simulink model "ecg_simulation"  (R2024b)
settings: Solver=VariableStepAuto  StartTime=0.0  StopTime=10.0  RelTol=1e-3
libraries: simulink x1

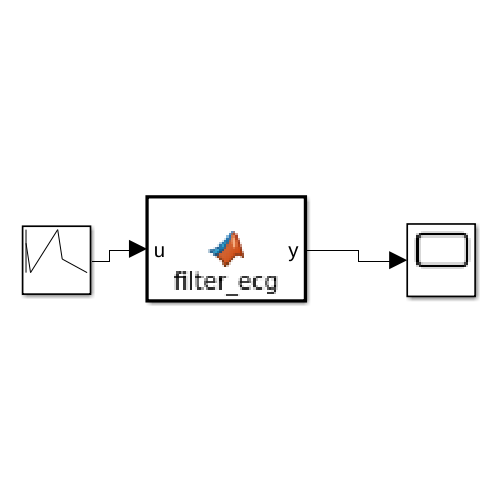
[thumbnail: Simulink's stored preview of the top-level diagram]
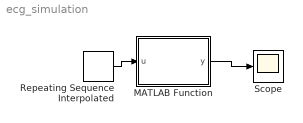
== system ecg_simulation ==
  MATLAB Function : MATLAB Function  TreatAsAtomicUnit=on
  Repeating Sequence Interpolated : simulink/Sources/Repeating Sequence Interpolated  OutValues=[3 1 4 2 1].'  TimeValues=[0 0.1 0.5 0.6 1].'  LookUpMeth=Interpolation-Use End Values  tsamp=0.01  OutMin=[]  OutMax=[]  OutDataTypeStr=double  OutputDataTypeScalingMode=double  OutDataType=fixdt(0,8)  OutScaling=2^-10
  Scope : Scope
  wires:
  Repeating Sequence Interpolated/1 -> MATLAB Function/1(u)
  MATLAB Function/1(y) -> Scope/1

== matlab function ecg_simulation/MATLAB Function ==
  data: u input; y output
function y = filter_ecg(u)
% فلترة إشارة ECG باستخدام bandpass من 0.5 Hz إلى 45 Hz

fs = 500; % تردد أخذ العينات
[b,a] = butter(2, [0.5 45]/(fs/2), 'bandpass');
y = filter(b, a, u); % الإشارة المفلترة
